simulink model "Instruction_memory"  (R2021a)
settings: Solver=VariableStepAuto  StartTime=0.0  StopTime=10.0  RelTol=1e-3
settings Model: Creator=kbhar  LastModifiedBy=kbhar

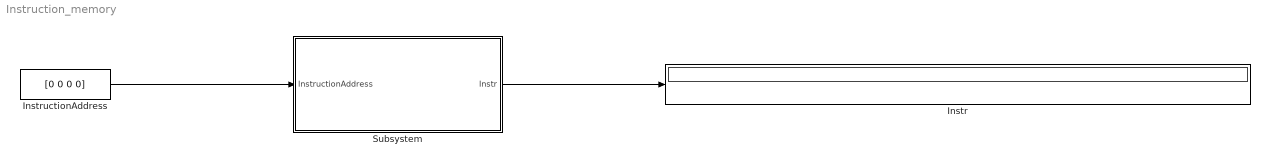
== system Instruction_memory ==
  Instr : Display
  InstructionAddress : Constant  Value=[0 0 0 0]
  Subsystem : Subsystem
  wires:
  InstructionAddress/1 -> Subsystem/1(InstructionAddress)
  Subsystem/1(Instr) -> Instr/1

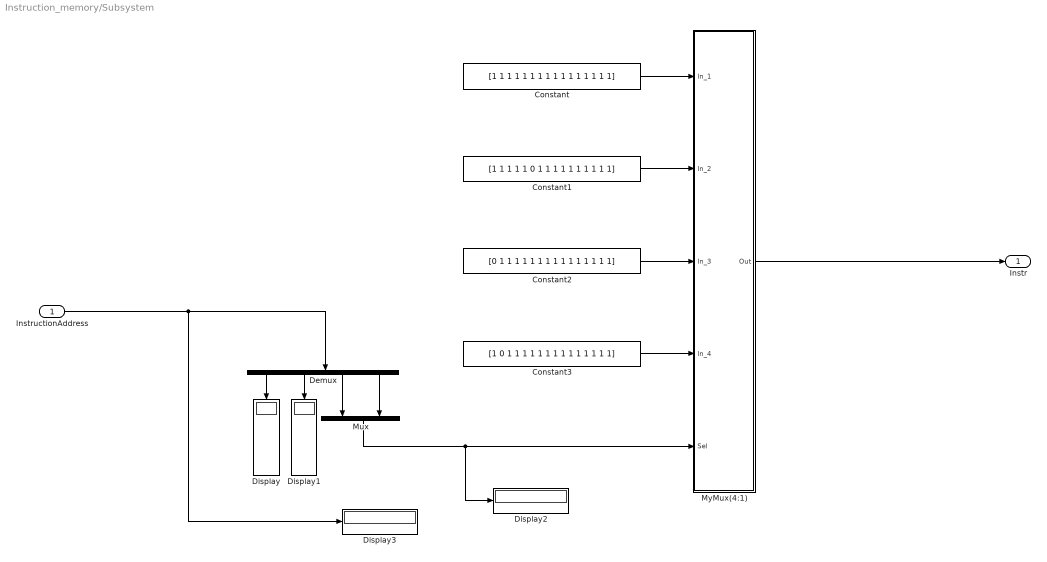
== system Instruction_memory/Subsystem ==
  InstructionAddress : Inport
  Constant : Constant  Value=[1 1 1 1 1 1 1 1 1 1 1 1 1 1 1 1]
  Constant1 : Constant  Value=[1 1 1 1 1 0 1 1 1 1 1 1 1 1 1 1]
  Constant2 : Constant  Value=[0 1 1 1 1 1 1 1 1 1 1 1 1 1 1 1]
  Constant3 : Constant  Value=[1 0 1 1 1 1 1 1 1 1 1 1 1 1 1 1]
  Demux : Demux
  Display{,1..3} (4 alike) : Display
  Mux : Mux  Inputs=2
  MyMux(4:1) : Subsystem
  Instr : Outport
  wires:
  Mux/1 -> Display2/1, MyMux(4:1)/5(Sel)
  Constant1/1 -> MyMux(4:1)/2(In_2)
  InstructionAddress/1 -> Display3/1, Demux/1
  Demux/4 -> Mux/2
  Constant2/1 -> MyMux(4:1)/3(In_3)
  Demux/1 -> Display/1
  Demux/3 -> Mux/1
  Demux/2 -> Display1/1
  Constant/1 -> MyMux(4:1)/1(In_1)
  Constant3/1 -> MyMux(4:1)/4(In_4)
  MyMux(4:1)/1(Out) -> Instr/1

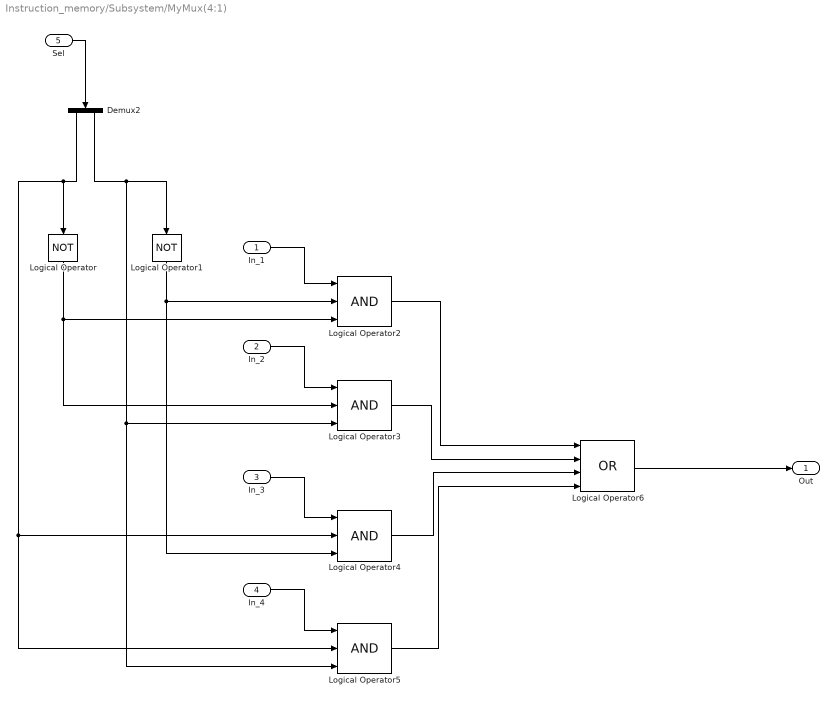
== system Instruction_memory/Subsystem/MyMux(4:1) ==
  In_1 : Inport
  In_2 : Inport  Port=2
  In_3 : Inport  Port=3
  In_4 : Inport  Port=4
  Sel : Inport  Port=5
  Demux2 : Demux  Outputs=2
  Logical Operator : Logic  Operator=NOT  AllPortsSameDT=off  OutDataTypeStr=boolean
  Logical Operator1 : Logic  Operator=NOT  AllPortsSameDT=off  OutDataTypeStr=boolean
  Logical Operator{2..5} (4 alike) : Logic  Inputs=3  AllPortsSameDT=off  OutDataTypeStr=boolean
  Logical Operator6 : Logic  Operator=OR  Inputs=4  AllPortsSameDT=off  OutDataTypeStr=boolean
  Out : Outport
  wires:
  Demux2/1 -> Logical Operator4/2, Logical Operator5/2, Logical Operator/1
  Demux2/2 -> Logical Operator5/3, Logical Operator3/3, Logical Operator1/1
  Logical Operator1/1 -> Logical Operator2/2, Logical Operator4/3
  Logical Operator2/1 -> Logical Operator6/1
  Logical Operator3/1 -> Logical Operator6/2
  Logical Operator/1 -> Logical Operator2/3, Logical Operator3/2
  Logical Operator4/1 -> Logical Operator6/3
  Logical Operator5/1 -> Logical Operator6/4
  In_2/1 -> Logical Operator3/1
  In_3/1 -> Logical Operator4/1
  In_4/1 -> Logical Operator5/1
  In_1/1 -> Logical Operator2/1
  Logical Operator6/1 -> Out/1
  Sel/1 -> Demux2/1
